simulink model "identifyOnHW"  (R2018b)
settings: Solver=FixedStepDiscrete  StartTime=0.0  StopTime=2500  FixedStep=0.005  RelTol=1e-3
settings Model: Creator=Bondi  LastModifiedBy=Bondi

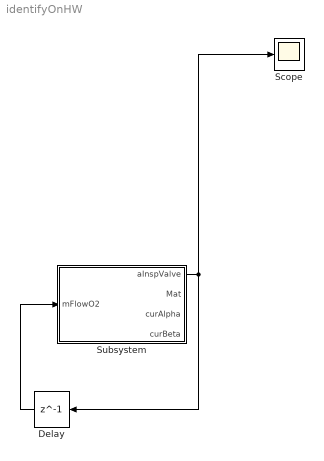
== system identifyOnHW ==
  Delay : Delay  DelayLength=1  InitialCondition=0
  Scope : Scope
  Subsystem : Subsystem
  wires:
  Subsystem/1(aInspValve) -> Delay/1, Scope/1
  Delay/1 -> Subsystem/1(mFlowO2)

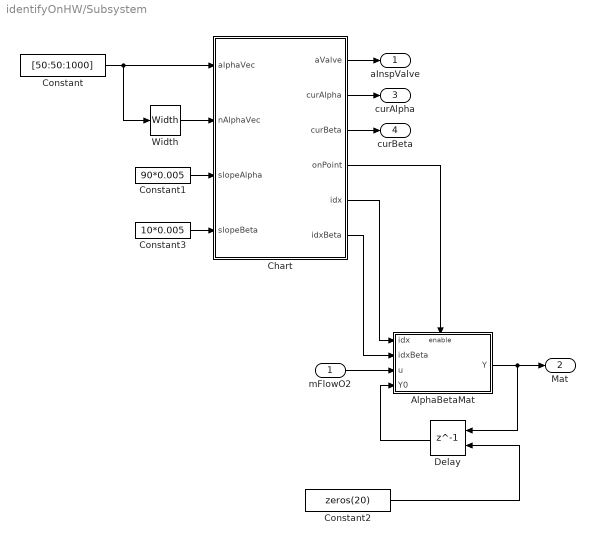
== system identifyOnHW/Subsystem ==
  mFlowO2 : Inport
  AlphaBetaMat : Subsystem
  Chart : Stateflow chart  TreatAsAtomicUnit=on
  Constant : Constant  Value=[50:50:1000]
  Constant1 : Constant  Value=90*0.005
  Constant2 : Constant  Value=zeros(20)
  Constant3 : Constant  Value=10*0.005
  Delay : Delay  DelayLength=1  InitialConditionSource=Input port
      settings: InputPortMap=u0,p4
  Width : Width
  aInspValve : Outport  OutputWhenDisabled=reset  InitialOutput=0
  Mat : Outport  Port=2  OutputWhenDisabled=reset  InitialOutput=0
  curAlpha : Outport  Port=3  OutputWhenDisabled=reset  InitialOutput=0
  curBeta : Outport  Port=4  OutputWhenDisabled=reset  InitialOutput=0
  wires:
  Constant/1 -> Width/1, Chart/1(alphaVec)
  Width/1 -> Chart/2(nAlphaVec)
  Constant1/1 -> Chart/3(slopeAlpha)
  Constant3/1 -> Chart/4(slopeBeta)
  Chart/2(curAlpha) -> curAlpha/1
  Chart/3(curBeta) -> curBeta/1
  Chart/4(onPoint) -> AlphaBetaMat/Enable
  Chart/5(idx) -> AlphaBetaMat/1(idx)
  Chart/6(idxBeta) -> AlphaBetaMat/2(idxBeta)
  AlphaBetaMat/1(Y) -> Delay/1, Mat/1
  Chart/1(aValve) -> aInspValve/1
  mFlowO2/1 -> AlphaBetaMat/3(u)
  Constant2/1 -> Delay/2
  Delay/1 -> AlphaBetaMat/4(Y0)

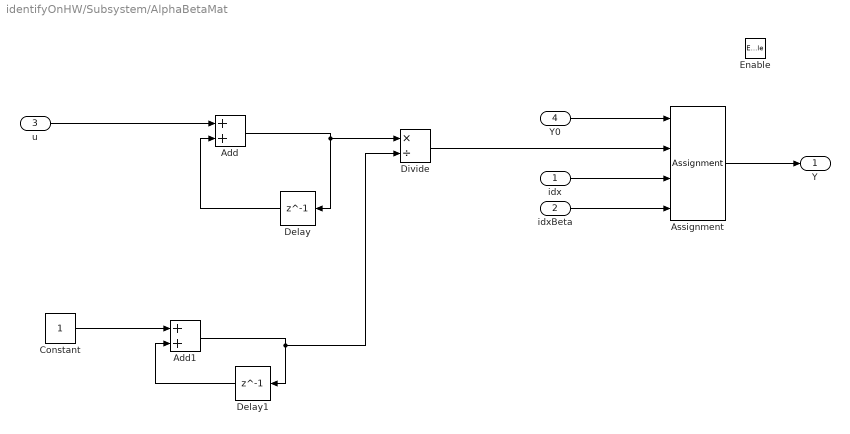
== system identifyOnHW/Subsystem/AlphaBetaMat ==
  idx : Inport
  idxBeta : Inport  Port=2
  u : Inport  Port=3
  Y0 : Inport  Port=4
  Enable : EnablePort  StatesWhenEnabling=reset
  Add : Sum
  Add1 : Sum
  Assignment : Assignment  NumberOfDimensions=2  DiagnosticForDimensions=Warning  IndexOptions=Index vector (port),Index vector (port)  Indices=1,1  OutputSizes=1,1
  Constant : Constant
  Delay : Delay  DelayLength=1
  Delay1 : Delay  DelayLength=1  InitialCondition=0
  Divide : Product  Inputs=*/  SaturateOnIntegerOverflow=on  RndMeth=Zero
  Y : Outport
  wires:
  idx/1 -> Assignment/3
  idxBeta/1 -> Assignment/4
  Assignment/1 -> Y/1
  Y0/1 -> Assignment/1
  Delay/1 -> Add/2
  Delay1/1 -> Add1/2
  Add1/1 -> Divide/2, Delay1/1
  Add/1 -> Divide/1, Delay/1
  u/1 -> Add/1
  Constant/1 -> Add1/1
  Divide/1 -> Assignment/2

== stateflow chart identifyOnHW/Subsystem/Chart ==
  state y
  state Initialize
  state RunAlphaValue
    en:
    curAlpha=alphaVec(idx)
    state RampToAlpha
      en:
      aValve=0;
      en,du:
      aValve=min(curAlpha,aValve+slopeAlpha)
    state Done
    state RampToBeta
      en:
      idxBeta=max(idxBeta,1);
      curBeta=alphaVec(idxBeta);
      en,du:
      aValve=max(curBeta,aValve-slopeBeta)
    state Hold
      en:
      onPoint=true;
      ex:
      onPoint=false;
    (default) -> RampToAlpha
    Hold -> Done [order 1] : [after(200,tick) && ...
        | idxBeta==1]
    RampToAlpha -> RampToBeta : [aValve>=curAlpha]
        | {idxBeta=idx}
    Hold -> RampToBeta [order 2] : [after(200,tick)]
        | {idxBeta=idxBeta-1;}
    RampToBeta -> Hold : [aValve<=curBeta]
  (default) -> Initialize
  (junction 16) -> y [order 2]
  Initialize -> RunAlphaValue : [after(200,tick)]
      | {idx=1;}
  (junction 16) -> (junction 17) [order 1] : [idx<nAlphaVec]
  RunAlphaValue -> (junction 16) : [in(RunAlphaValue.Done)]
  (junction 17) -> RunAlphaValue : {idx=idx+1;}
  data: aValve output; alphaVec input; nAlphaVec input; curAlpha output; curBeta output; onPoint output; idx output; idxBeta output; slopeAlpha input; slopeBeta input
